simulink model "EML_Example_QNX"  (R2017a)
settings: Solver=FixedStepAuto  StartTime=0.0  StopTime=10.0  RelTol=1e-3  EnableMultiTasking=on
settings Model: Creator=darenlee  LastModifiedBy=darenlee
settings SolverCC: PositivePriorityOrder=on
settings OptimizationCC: UseSpecifiedMinMax=on  ZeroExternalMemoryAtStartup=off  ZeroInternalMemoryAtStartup=off  EfficientFloat2IntCast=on  LifeSpan=1  MaxStackSize=64
settings DebuggingCC: SFUnexpectedBacktrackingDiag=warning  SFNoUnconditionalDefaultTransitionDiag=warning  SFExecutionAtInitializationDiag=none
settings SFSimCC: SimCustomHeaderCode="#include \"external_include_file.h\""  SimUserSources=external_src_file.c  MATLABDynamicMemAlloc=off
settings RTWCC: SystemTargetFile=ert.tlc  HardwareBoard=QNX-x86  TLCOptions="-aInlineSetEventsForThisBaseRateFcn=TLC_FALSE -aSuppressMultiTaskScheduler=TLC_FALSE  -aRateBasedStepFcn=0"  TemplateMakefile=ert_default_tmf  Description=Embedded Coder  GenerateReport=on  Toolchain=QNX QCC Toolchain  IncludeHyperlinkInReport=on  LaunchReport=on  GenerateTraceInfo=on  GenerateTraceReport=on  GenerateTraceReportSl=on  GenerateTraceReportSf=on  GenerateTraceReportEml=on
settings CodeAppCC: ForceParamTrailComments=on  IgnoreCustomStorageClasses=off  OperatorAnnotations=on  SimulinkDataObjDesc=on  SFDataObjDesc=on  MATLABFcnDesc=on  InsertBlockDesc=on  MATLABSourceComments=on
settings ERTTargetCC: UtilityFuncGeneration=Shared location  MultiwordLength=2048  CombineSignalStateStructs=on
settings ConfigComp: CovMetricSettings=dw  CovHtmlReporting=on  CovSaveCumulativeToWorkspaceVar=on  CovSaveSingleToWorkspaceVar=on  CovExternalEMLEnable=off

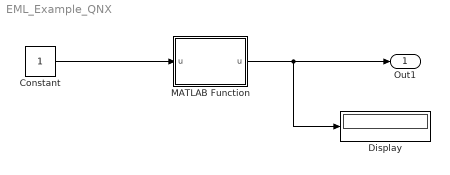
== system EML_Example_QNX ==
  Constant : Constant  SampleTime=1
  Display : Display
  MATLAB Function : MATLAB Function  TreatAsAtomicUnit=on
  Out1 : Outport
  wires:
  Constant/1 -> MATLAB Function/1("u ")
  MATLAB Function/1(u) -> Display/1, Out1/1

== matlab function EML_Example_QNX/MATLAB Function ==
  data: u input; u output
function u = fcn(u)
%#codegen
persistent state1


if isempty(state1)
    % This can be used as a way to initialize the states that exist
    % within the block
    state1 = -10;
    if coder.target('rtw')            
        coder.updateBuildInfo('addSourceFiles','external_src_file.c');
        coder.updateBuildInfo('addIncludeFiles','external_include_file.h');

        coder.ceval('call_this_at_the_very_first_time_step');
    end
end

if coder.target('rtw') 
    %This is for code generation. Code you write in this if branch will
    %show up in the generated code only
    
%     y = 0; %sometimes you need to pre-define your output like this
    coder.ceval('external_function',coder.ref(u));
    
    str_msg1 = ['Value of the output is = %f', uint8(10), uint8(0)];
    coder.ceval('printf',coder.rref(str_msg1),u);
    
    str_msg2 = ['state1 = %f', uint8(10), uint8(0)];
    coder.ceval('printf', coder.rref(str_msg2),state1);
    
else
    %this is for simulation only
    u = u*2;


end

state1 =  state1 + 1;

end
